simulink model "Vehicle_Dynamics_Tests"  (R2013b)
settings: Solver=ode15s  StartTime=0.0  StopTime=10  MaxStep=0.01  RelTol=1e-4  AbsTol=1e-4
PostLoadFcn:
  | Configure_TNO_Tire_Test('handling');
undefined symbols (not defined in the file or in its folder): angparking, delta, is, TNO_Veh_PARAM, tparking, tswd, tvxset, vxset, X, Y, Z
libraries: sm_lib x53, nesl_utility x25, Delft_Tyre_sm2glib x16
(part 1 of 2)
Description:
  | Copyright 2013 The MathWorks, Inc.
settings Model: Creator=smiller  LastModifiedBy=hofstadrhmtvd
settings DataIOCC: LimitDataPoints=off  SaveOutput=off  OutputTimes=[0:0.01:10]
settings OptimizationCC: ExpressionDepthLimit=2147483647
settings DebuggingCC: StateNameClashWarn=warning
settings ConfigurationSet: Description=SimMechanics 2G
settings ExplorerConfigSet: InternalSimMechanicsExplorerSettings="<ExplorerConfiguration><canonicalview>default</canonicalview><TilePanel><TileInfo><Tiles Columns=\"1\" Count=\"1\" Rows=\"1\"><Column Left=\"2\" Weight=\"1\"/><Column Left=\"786\"/><Row Top=\"2\" Weight=\"1\"/><Row Top=\"392\"/><Tile Height=\"1\" Width=\"1\" X=\"0\" Y=\"0\"/></Tiles></TileInfo><SceneInfo><SceneViewer><BGColor><R>0.80000001192092896</R><G>0.80000001192092896</G><B>0.80000001192092896</B></BGColor><Camera><Position><X>5.6749032986341916</X><Y>0.8952491746014456</Y><Z>0.76840563569508813</Z></Position><Center><X>-1.5032858848571777</X><Y>0.8952491746014456</Y><Z>0.76840563569508813</Z></Center><Up><X>-0</X><Y>0</Y><Z>1</Z></Up><Left>-1.4372989570944883</Left><Right>1.4372989570944883</Right><Bottom>-1.1681998313418454</Bottom><Top>1.1681998313418454</Top></Camera></SceneViewer></SceneInfo></TilePanel></ExplorerConfiguration>"

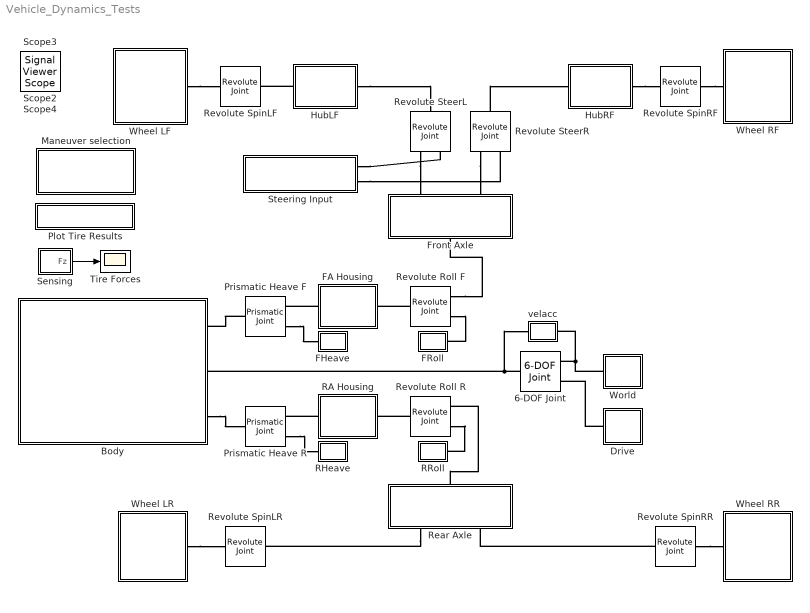
== system Vehicle_Dynamics_Tests ==
  6-DOF Joint : sm_lib/Joints/6-DOF Joint  SenseConstraintForceX=off  SenseConstraintForceY=off  SenseConstraintForceZ=off  SenseConstraintTorqueX=off  SenseConstraintTorqueY=off  SenseConstraintTorqueZ=off  ConstraintWrenchDir=FollowerOnBase  ConstraintWrenchFrame=BaseFrame  PxEquilibriumPosition=0  PxEquilibriumPositionUnits=m  PxSpringStiffness=0  PxSpringStiffnessUnits=N/m  PxDampingCoefficient=0  PxDampingCoefficientUnits=N/(m/s)  PxTorqueActuationMode=InputTorque  PxMotionActuationMode=ComputedMotion  PxSensePosition=off  PxSenseVelocity=off  PxSenseAcceleration=off  PxSenseTorqueForce=off  PxPositionTargetValue=0  PxPositionTargetValueUnits=m  PxPositionTargetSpecify=off  PxPositionTargetPriority=High  PxVelocityTargetValue=TNO_Veh_PARAM.InitVel.Vehicle  PxVelocityTargetValueUnits=m/s  PxVelocityTargetSpecify=on  PxVelocityTargetPriority=High  PyEquilibriumPosition=0  PyEquilibriumPositionUnits=m  PySpringStiffness=0  PySpringStiffnessUnits=N/m  PyDampingCoefficient=0  PyDampingCoefficientUnits=N/(m/s)  PyTorqueActuationMode=NoTorque  PyMotionActuationMode=ComputedMotion  PySensePosition=off  PySenseVelocity=off  PySenseAcceleration=off  PySenseTorqueForce=off  PyPositionTargetValue=0  PyPositionTargetValueUnits=m  PyPositionTargetSpecify=off  PyPositionTargetPriority=High  PyVelocityTargetValue=0  PyVelocityTargetValueUnits=m/s  PyVelocityTargetSpecify=off  PyVelocityTargetPriority=High  PzEquilibriumPosition=0  PzEquilibriumPositionUnits=m  PzSpringStiffness=0  PzSpringStiffnessUnits=N/m  PzDampingCoefficient=0  PzDampingCoefficientUnits=N/(m/s)  PzTorqueActuationMode=NoTorque  PzMotionActuationMode=ComputedMotion  PzSensePosition=off  PzSenseVelocity=off  PzSenseAcceleration=off  PzSenseTorqueForce=off  PzPositionTargetValue=0  PzPositionTargetValueUnits=m  PzPositionTargetSpecify=off  PzPositionTargetPriority=High  PzVelocityTargetValue=0  PzVelocityTargetValueUnits=m/s  PzVelocityTargetSpecify=off  PzVelocityTargetPriority=High  SphDefPosRotationMethod=None  SphDefPosRotationAngleUnits=deg  SphDefPosRotationStandardAxis=+Z  SphDefPosRotationAngle=0  SphDefPosRotationArbitraryAxis=[0 0 1]  SphDefPosFollAlignAxisA=+X  SphDefPosBaseAlignAxisA=+Y  SphDefPosFollAlignAxisB=+Y  SphDefPosBaseAlignAxisB=+Z  SphEqPosRotationMethod=None  SphEqPosRotationAngleUnits=deg  SphEqPosRotationStandardAxis=+Z  SphEqPosRotationAngle=0  SphEqPosRotationArbitraryAxis=[0 0 1]  SphEqPosFollAlignAxisA=+X  SphEqPosBaseAlignAxisA=+Y  SphEqPosFollAlignAxisB=+Y  SphEqPosBaseAlignAxisB=+Z  SphSpringStiffness=0  SphSpringStiffnessUnits=N*m/deg  SphDampingCoefficient=0  SphDampingCoefficientUnits=N*m/(deg/s)  SphActuateTorqueX=off  SphActuateTorqueY=off  SphActuateTorqueZ=off  SphActuateTorque=off  SphTorqueActuationMode=NoTorque  SphMotionActuationMode=ComputedMotion  SphActuationFrame=BaseFrame  SphSensePosition=off  SphSenseVelocityX=off  SphSenseVelocityY=off  SphSenseVelocityZ=off  SphSenseVelocity=off  SphSenseAccelerationX=off  SphSenseAccelerationY=off  SphSenseAccelerationZ=off  SphSenseAcceleration=off  SphSenseTorqueX=off  SphSenseTorqueY=off  SphSenseTorqueZ=off  SphSenseTorqueForce=off  SphSensingFrame=BaseFrame  SphPositionTargetRotationMethod=None  SphPositionTargetRotationAngleUnits=deg  SphPositionTargetRotationStandardAxis=+Z  SphPositionTargetRotationAngle=0  SphPositionTargetRotationArbitraryAxis=[0 0 1]  SphPositionTargetFollAlignAxisA=+X  SphPositionTargetBaseAlignAxisA=+Y  SphPositionTargetFollAlignAxisB=+Y  SphPositionTargetBaseAlignAxisB=+Z  SphPositionTargetSpecify=off  SphPositionTargetPriority=High  SphVelocityTargetValue=[0 0 0]  SphVelocityTargetValueUnits=deg/s  SphVelocityTargetSpecify=off  SphVelocityTargetPriority=High  SphVelocityTargetInFollowerFrame=on  BlockFunction=simmechanics.library.joints.sixdof_joint
  Body : Subsystem
      mask Display: image('VehicleBody.png')
  Drive : Subsystem
  FA Housing : Subsystem
  FHeave : Subsystem
      mask Display: disp('FHe');
  FRoll : Subsystem
      mask Display: disp('FRo');
  Front Axle : Subsystem
  HubLF : Subsystem
  HubRF : Subsystem
  Maneuver selection : Subsystem  mask{maneuver_type=Slalom}
      mask prompts: maneuver_type "Maneuver choice"
      mask init:
      | if strcmp(maneuver_type,'Slalom')
      |     Configure_TNO_Tire_Test('slalom');
      | elseif strcmp(maneuver_type,'4 Post Testrig')
      |     Configure_TNO_Tire_Test('4poster');
      | elseif strcmp(maneuver_type,'Parking')
      |     Configure_TNO_Tire_Test('parking');
      | elseif strcmp(maneuver_type,'Ride')
      |     Configure_TNO_Tire_Test('ride');
      | elseif strcmp(maneuver_type,'Step Steer')
      |     Configure_TNO_Tire_Test('handling');
      | elseif strcmp(maneuver_type,'Sine with Dwell')
      |     Configure_TNO_Tire_Test('sinewithdwell');
      | end
      mask TypeOptions maneuver_type: Slalom | 4 Post Testrig | Parking | Ride | Step Steer | Sine with Dwell
      mask DialogControl Update_Diagram Prompt: Update Diagram
      mask DialogControl Update_Diagram Callback: set_param(bdroot,'SimulationCommand','Update')
      mask Display:
      | fprintf('Maneuver:\n\n')
      | fprintf(maneuver_type);
  Plot Tire Results : Subsystem
      settings: OpenFcn=PlotTireOutputs_UI
      mask Display: disp('Plot Tire Results');
  Prismatic Heave F : sm_lib/Joints/Prismatic Joint  SenseConstraintForceX=off  SenseConstraintForceY=off  SenseConstraintForceZ=off  SenseConstraintTorqueX=off  SenseConstraintTorqueY=off  SenseConstraintTorqueZ=off  ConstraintWrenchDir=FollowerOnBase  ConstraintWrenchFrame=BaseFrame  EquilibriumPosition=TNO_Veh_PARAM.Suspension.FA.Heave.EqPos  EquilibriumPositionUnits=m  SpringStiffness=TNO_Veh_PARAM.Suspension.FA.Heave.Stiffness  SpringStiffnessUnits=N/m  DampingCoefficient=TNO_Veh_PARAM.Suspension.FA.Heave.Damping  DampingCoefficientUnits=N/(m/s)  TorqueActuationMode=NoTorque  MotionActuationMode=ComputedMotion  SensePosition=on  SenseVelocity=off  SenseAcceleration=off  SenseTorqueForce=off  PositionTargetValue=0  PositionTargetValueUnits=m  PositionTargetSpecify=off  PositionTargetPriority=High  VelocityTargetValue=0  VelocityTargetValueUnits=m/s  VelocityTargetSpecify=off  VelocityTargetPriority=High  BlockFunction=simmechanics.library.joints.prismatic_joint
  Prismatic Heave R : sm_lib/Joints/Prismatic Joint  SenseConstraintForceX=off  SenseConstraintForceY=off  SenseConstraintForceZ=off  SenseConstraintTorqueX=off  SenseConstraintTorqueY=off  SenseConstraintTorqueZ=off  ConstraintWrenchDir=FollowerOnBase  ConstraintWrenchFrame=BaseFrame  EquilibriumPosition=TNO_Veh_PARAM.Suspension.RA.Heave.EqPos  EquilibriumPositionUnits=m  SpringStiffness=TNO_Veh_PARAM.Suspension.RA.Heave.Stiffness  SpringStiffnessUnits=N/m  DampingCoefficient=TNO_Veh_PARAM.Suspension.RA.Heave.Damping  DampingCoefficientUnits=N/(m/s)  TorqueActuationMode=NoTorque  MotionActuationMode=ComputedMotion  SensePosition=on  SenseVelocity=off  SenseAcceleration=off  SenseTorqueForce=off  PositionTargetValue=0  PositionTargetValueUnits=m  PositionTargetSpecify=off  PositionTargetPriority=High  VelocityTargetValue=0  VelocityTargetValueUnits=m/s  VelocityTargetSpecify=off  VelocityTargetPriority=High  BlockFunction=simmechanics.library.joints.prismatic_joint
  RA Housing : Subsystem
  RHeave : Subsystem
      mask Display: disp('RHe')
  RRoll : Subsystem
      mask Display: disp('RRo');
  Rear Axle : Subsystem
  Revolute SpinLF : sm_lib/Joints/Revolute Joint  SenseConstraintForceX=off  SenseConstraintForceY=off  SenseConstraintForceZ=off  SenseConstraintTorqueX=off  SenseConstraintTorqueY=off  SenseConstraintTorqueZ=off  ConstraintWrenchDir=FollowerOnBase  ConstraintWrenchFrame=BaseFrame  EquilibriumPosition=0  EquilibriumPositionUnits=rad  SpringStiffness=0  SpringStiffnessUnits=N*m/rad  DampingCoefficient=0  DampingCoefficientUnits=N*m/(rad/s)  TorqueActuationMode=NoTorque  MotionActuationMode=ComputedMotion  SensePosition=off  SenseVelocity=off  SenseAcceleration=off  SenseTorqueForce=off  PositionTargetValue=0  PositionTargetValueUnits=deg  PositionTargetSpecify=off  PositionTargetPriority=High  VelocityTargetValue=TNO_Veh_PARAM.InitVel.LF  VelocityTargetValueUnits=rad/s  VelocityTargetSpecify=on  VelocityTargetPriority=High  BlockFunction=simmechanics.library.joints.revolute_joint
  Revolute SpinLR : sm_lib/Joints/Revolute Joint  SenseConstraintForceX=off  SenseConstraintForceY=off  SenseConstraintForceZ=off  SenseConstraintTorqueX=off  SenseConstraintTorqueY=off  SenseConstraintTorqueZ=off  ConstraintWrenchDir=FollowerOnBase  ConstraintWrenchFrame=BaseFrame  EquilibriumPosition=0  EquilibriumPositionUnits=rad  SpringStiffness=0  SpringStiffnessUnits=N*m/rad  DampingCoefficient=0  DampingCoefficientUnits=N*m/(rad/s)  TorqueActuationMode=NoTorque  MotionActuationMode=ComputedMotion  SensePosition=off  SenseVelocity=off  SenseAcceleration=off  SenseTorqueForce=off  PositionTargetValue=0  PositionTargetValueUnits=deg  PositionTargetSpecify=off  PositionTargetPriority=High  VelocityTargetValue=TNO_Veh_PARAM.InitVel.LR  VelocityTargetValueUnits=rad/s  VelocityTargetSpecify=on  VelocityTargetPriority=High  BlockFunction=simmechanics.library.joints.revolute_joint
  Revolute SpinRF : sm_lib/Joints/Revolute Joint  SenseConstraintForceX=off  SenseConstraintForceY=off  SenseConstraintForceZ=off  SenseConstraintTorqueX=off  SenseConstraintTorqueY=off  SenseConstraintTorqueZ=off  ConstraintWrenchDir=FollowerOnBase  ConstraintWrenchFrame=BaseFrame  EquilibriumPosition=0  EquilibriumPositionUnits=rad  SpringStiffness=0  SpringStiffnessUnits=N*m/rad  DampingCoefficient=0  DampingCoefficientUnits=N*m/(rad/s)  TorqueActuationMode=NoTorque  MotionActuationMode=ComputedMotion  SensePosition=off  SenseVelocity=off  SenseAcceleration=off  SenseTorqueForce=off  PositionTargetValue=0  PositionTargetValueUnits=deg  PositionTargetSpecify=off  PositionTargetPriority=High  VelocityTargetValue=TNO_Veh_PARAM.InitVel.RF  VelocityTargetValueUnits=rad/s  VelocityTargetSpecify=on  VelocityTargetPriority=High  BlockFunction=simmechanics.library.joints.revolute_joint
  Revolute SpinRR : sm_lib/Joints/Revolute Joint  SenseConstraintForceX=off  SenseConstraintForceY=off  SenseConstraintForceZ=off  SenseConstraintTorqueX=off  SenseConstraintTorqueY=off  SenseConstraintTorqueZ=off  ConstraintWrenchDir=FollowerOnBase  ConstraintWrenchFrame=BaseFrame  EquilibriumPosition=0  EquilibriumPositionUnits=rad  SpringStiffness=0  SpringStiffnessUnits=N*m/rad  DampingCoefficient=0  DampingCoefficientUnits=N*m/(rad/s)  TorqueActuationMode=NoTorque  MotionActuationMode=ComputedMotion  SensePosition=off  SenseVelocity=off  SenseAcceleration=off  SenseTorqueForce=off  PositionTargetValue=0  PositionTargetValueUnits=deg  PositionTargetSpecify=off  PositionTargetPriority=High  VelocityTargetValue=TNO_Veh_PARAM.InitVel.RR  VelocityTargetValueUnits=rad/s  VelocityTargetSpecify=on  VelocityTargetPriority=High  BlockFunction=simmechanics.library.joints.revolute_joint
  Revolute SteerL : sm_lib/Joints/Revolute Joint  SenseConstraintForceX=off  SenseConstraintForceY=off  SenseConstraintForceZ=off  SenseConstraintTorqueX=off  SenseConstraintTorqueY=off  SenseConstraintTorqueZ=off  ConstraintWrenchDir=FollowerOnBase  ConstraintWrenchFrame=BaseFrame  EquilibriumPosition=0  EquilibriumPositionUnits=rad  SpringStiffness=0  SpringStiffnessUnits=N*m/rad  DampingCoefficient=0  DampingCoefficientUnits=N*m/(rad/s)  TorqueActuationMode=ComputedTorque  MotionActuationMode=InputMotion  SensePosition=off  SenseVelocity=off  SenseAcceleration=off  SenseTorqueForce=off  PositionTargetValue=0  PositionTargetValueUnits=deg  PositionTargetSpecify=off  PositionTargetPriority=High  VelocityTargetValue=66  VelocityTargetValueUnits=rad/s  VelocityTargetSpecify=off  VelocityTargetPriority=High  BlockFunction=simmechanics.library.joints.revolute_joint
  Revolute SteerR : sm_lib/Joints/Revolute Joint  SenseConstraintForceX=off  SenseConstraintForceY=off  SenseConstraintForceZ=off  SenseConstraintTorqueX=off  SenseConstraintTorqueY=off  SenseConstraintTorqueZ=off  ConstraintWrenchDir=FollowerOnBase  ConstraintWrenchFrame=BaseFrame  EquilibriumPosition=0  EquilibriumPositionUnits=rad  SpringStiffness=0  SpringStiffnessUnits=N*m/rad  DampingCoefficient=0  DampingCoefficientUnits=N*m/(rad/s)  TorqueActuationMode=ComputedTorque  MotionActuationMode=InputMotion  SensePosition=off  SenseVelocity=off  SenseAcceleration=off  SenseTorqueForce=off  PositionTargetValue=0  PositionTargetValueUnits=deg  PositionTargetSpecify=off  PositionTargetPriority=High  VelocityTargetValue=66  VelocityTargetValueUnits=rad/s  VelocityTargetSpecify=off  VelocityTargetPriority=High  BlockFunction=simmechanics.library.joints.revolute_joint
  Revolute Roll F : sm_lib/Joints/Revolute Joint  SenseConstraintForceX=off  SenseConstraintForceY=off  SenseConstraintForceZ=off  SenseConstraintTorqueX=off  SenseConstraintTorqueY=off  SenseConstraintTorqueZ=off  ConstraintWrenchDir=FollowerOnBase  ConstraintWrenchFrame=BaseFrame  EquilibriumPosition=0  EquilibriumPositionUnits=rad  SpringStiffness=TNO_Veh_PARAM.Suspension.FA.Roll.Stiffness  SpringStiffnessUnits=N*m/rad  DampingCoefficient=TNO_Veh_PARAM.Suspension.FA.Roll.Damping  DampingCoefficientUnits=N*m/(rad/s)  TorqueActuationMode=NoTorque  MotionActuationMode=ComputedMotion  SensePosition=on  SenseVelocity=off  SenseAcceleration=off  SenseTorqueForce=off  PositionTargetValue=0  PositionTargetValueUnits=deg  PositionTargetSpecify=off  PositionTargetPriority=High  VelocityTargetValue=0  VelocityTargetValueUnits=deg/s  VelocityTargetSpecify=off  VelocityTargetPriority=High  BlockFunction=simmechanics.library.joints.revolute_joint
  Revolute Roll R : sm_lib/Joints/Revolute Joint  SenseConstraintForceX=off  SenseConstraintForceY=off  SenseConstraintForceZ=off  SenseConstraintTorqueX=off  SenseConstraintTorqueY=off  SenseConstraintTorqueZ=off  ConstraintWrenchDir=FollowerOnBase  ConstraintWrenchFrame=BaseFrame  EquilibriumPosition=0  EquilibriumPositionUnits=rad  SpringStiffness=TNO_Veh_PARAM.Suspension.RA.Roll.Stiffness  SpringStiffnessUnits=N*m/rad  DampingCoefficient=TNO_Veh_PARAM.Suspension.RA.Roll.Damping  DampingCoefficientUnits=N*m/(rad/s)  TorqueActuationMode=NoTorque  MotionActuationMode=ComputedMotion  SensePosition=on  SenseVelocity=off  SenseAcceleration=off  SenseTorqueForce=off  PositionTargetValue=0  PositionTargetValueUnits=deg  PositionTargetSpecify=off  PositionTargetPriority=High  VelocityTargetValue=0  VelocityTargetValueUnits=deg/s  VelocityTargetSpecify=off  VelocityTargetPriority=High  BlockFunction=simmechanics.library.joints.revolute_joint
  Sensing : Subsystem
  Steering Input : Subsystem  Variant=on  OverrideUsingVariant=Slalom
  Tire Forces : Scope
      settings: YMin=3500  YMax=6000
  Wheel LF : Subsystem
      mask Display: image('WheelL.png')
  Wheel LR : Subsystem
      mask Display: image('WheelL.png')
  Wheel RF : Subsystem
      mask Display: image('WheelR.png')
  Wheel RR : Subsystem
      mask Display: image('WheelR.png')
  World : Subsystem
  velacc : Subsystem
      mask Display: disp('va')
  Scope2 : SignalViewerScope  IOType=viewer  RefreshTime=0.035000
  Scope3 : SignalViewerScope  IOType=viewer  ZoomMode=yonly  LegendLocations="0.77309     0.66156     0.17615     0.19796"  RefreshTime=0.035000
      settings: ShowLegends=on
  Scope4 : SignalViewerScope  IOType=viewer  RefreshTime=0.035000
      settings: SaveName=ScopeData2
  wires:
  Sensing/1(Fz) -> Tire Forces/1
  connections:
  6-DOF Joint/RConn1 -- velacc/RConn1 -- Body/LConn2
  World/LConn1 -- velacc/LConn1 -- 6-DOF Joint/LConn1
  Rear Axle/RConn1 -- Revolute SpinLR/LConn1
  Revolute SteerR/LConn1 -- Front Axle/RConn2
  Revolute SteerL/LConn1 -- Front Axle/RConn1
  Steering Input/RConn1 -- Revolute SteerL/LConn2
  Prismatic Heave F/LConn1 -- Body/LConn1
  Revolute Roll F/RConn1 -- Front Axle/LConn1
  Revolute Roll R/LConn1 -- RA Housing/RConn1
  Rear Axle/LConn1 -- Revolute Roll R/RConn1
  Body/LConn3 -- Prismatic Heave R/LConn1
  RA Housing/LConn1 -- Prismatic Heave R/RConn1
  FA Housing/LConn1 -- Prismatic Heave F/RConn1
  Revolute Roll F/LConn1 -- FA Housing/RConn1
  Prismatic Heave F/RConn2 -- FHeave/RConn1
  Revolute Roll F/RConn2 -- FRoll/RConn1
  Prismatic Heave R/RConn2 -- RHeave/LConn1
  Revolute Roll R/RConn2 -- RRoll/RConn1
  HubLF/LConn1 -- Revolute SteerL/RConn1
  HubLF/RConn1 -- Revolute SpinLF/LConn1
  HubRF/RConn1 -- Revolute SpinRF/LConn1
  Revolute SpinRF/RConn1 -- Wheel RF/LConn1
  Revolute SpinRR/RConn1 -- Wheel RR/LConn1
  Wheel LR/RConn1 -- Revolute SpinLR/RConn1
  Wheel LF/RConn1 -- Revolute SpinLF/RConn1
  Revolute SteerR/RConn1 -- HubRF/LConn1
  Revolute SpinRR/LConn1 -- Rear Axle/RConn2
  Steering Input/RConn2 -- Revolute SteerR/LConn2
  Drive/LConn1 -- 6-DOF Joint/LConn2

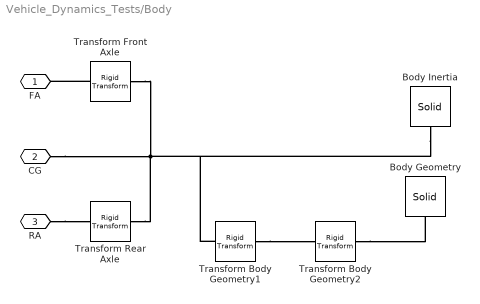
== system Vehicle_Dynamics_Tests/Body ==
  Body Geometry : sm_lib/Body Elements/Solid  InertiaType=Custom  Mass=0  MassUnits=kg  CenterOfMass=[0 0 0]  CenterOfMassUnits=m  MomentsOfInertia=[0 0 0]  MomentsOfInertiaUnits=kg*m^2  ProductsOfInertia=[0 0 0]  ProductsOfInertiaUnits=kg*m^2  DensityBased=on  Density=1000  DensityUnits=kg/(m^3)  GraphicType=FromGeometry  MarkerShape=Sphere  MarkerSize=10  MarkerSizeUnits=m  GraphicVisPropType=SimpleVisualProperties  GraphicDiffuseColor=[0.6 0.8 1.0]  GraphicSpecularColor=[0.5 0.5 0.5 1.0]  GraphicAmbientColor=[0.15 0.15 0.15 1.0]  GraphicEmissiveColor=[0.0 0.0 0.0 1.0]  GraphicShininess=75  GraphicOpacity=1  GeometryShape=FromFile  RectangleSize=[1 1]  RectangleSizeUnits=m  BrickDimensions=TNO_Veh_PARAM.Body.LWH  BrickDimensionUnits=m  CylinderRadius=1  CylinderRadiusUnits=m  CylinderLength=1  CylinderLengthUnits=m  SphereRadius=1  SphereRadiusUnits=m  EllipsoidRadii=[1 1 1]  EllipsoidRadiiUnits=m  ExtrusionCrossSection=[1 1; -1 1; -1 -1; 1 -1]  ExtrusionCrossSectionUnits=m  ExtrusionLength=1  ExtrusionLengthUnits=m  PolygonNumSides=3  PolygonOuterRadius=1  PolygonOuterRadiusUnits=m  ExtGeomFileName=VehicleBody.STL  ExtGeomFileUnits=mm  RevolutionCrossSection=[1 1; 1 -1; 2 -1; 2 1]  RevolutionCrossSectionUnits=m  RevolutionExtent=Full  RevolutionAngle=180  RevolutionAngleUnits=deg  BlockFunction=simmechanics.library.body_elements.solid
  Body Inertia : sm_lib/Body Elements/Solid  InertiaType=Custom  Mass=TNO_Veh_PARAM.Body.Mass  MassUnits=kg  CenterOfMass=[0 0 0]  CenterOfMassUnits=m  MomentsOfInertia=TNO_Veh_PARAM.Body.Inertias  MomentsOfInertiaUnits=kg*m^2  ProductsOfInertia=[0 0 0]  ProductsOfInertiaUnits=kg*m^2  DensityBased=on  Density=1000  DensityUnits=kg/(m^3)  GraphicType=FromGeometry  MarkerShape=Sphere  MarkerSize=10  MarkerSizeUnits=m  GraphicVisPropType=SimpleVisualProperties  GraphicDiffuseColor=[0.4 0.6 1.0]  GraphicSpecularColor=[0.5 0.5 0.5 1.0]  GraphicAmbientColor=[0.15 0.15 0.15 1.0]  GraphicEmissiveColor=[0.0 0.0 0.0 1.0]  GraphicShininess=75  GraphicOpacity=1.0  GeometryShape=Brick  RectangleSize=[1 1]  RectangleSizeUnits=m  BrickDimensions=TNO_Veh_PARAM.Body.LWH  BrickDimensionUnits=m  CylinderRadius=1  CylinderRadiusUnits=m  CylinderLength=1  CylinderLengthUnits=m  SphereRadius=1  SphereRadiusUnits=m  EllipsoidRadii=[1 1 1]  EllipsoidRadiiUnits=m  ExtrusionCrossSection=[1 1; -1 1; -1 -1; 1 -1]  ExtrusionCrossSectionUnits=m  ExtrusionLength=1  ExtrusionLengthUnits=m  PolygonNumSides=3  PolygonOuterRadius=1  PolygonOuterRadiusUnits=m  ExtGeomFileName=L:\PhysModDevTeamProject\MF_Tyre_64b\Demos\SimMechanics_demos\CadImportFiles\BMW M3-IGS - Imported1-1.STL  ExtGeomFileUnits=mm  RevolutionCrossSection=[1 1; 1 -1; 2 -1; 2 1]  RevolutionCrossSectionUnits=m  RevolutionExtent=Full  RevolutionAngle=180  RevolutionAngleUnits=deg  BlockFunction=simmechanics.library.body_elements.solid
  Transform Front Axle : sm_lib/Frames and Transforms/Rigid Transform  TranslationMethod=Cartesian  TranslationLengthUnit=m  TranslationStandardAxis=+Z  TranslationStandardOffset=0  TranslationCartesianOffset=[TNO_Veh_PARAM.Body.Length/2 0 -TNO_Veh_PARAM.Suspension.FA.Heave.Height]  TranslationROffset=0  TranslationROffsetUnits=m  TranslationZOffset=0  TranslationZOffsetUnits=m  TranslationThetaOffset=0  TranslationThetaOffsetUnits=deg  RotationMethod=None  RotationAngleUnits=deg  RotationStandardAxis=+Z  RotationAngle=0  RotationArbitraryAxis=[0 0 1]  FollAlignAxisA=+X  BaseAlignAxisA=+Y  FollAlignAxisB=+Y  BaseAlignAxisB=+Z  BlockFunction=simmechanics.library.frames_transforms.rigid_transform
  Transform Rear Axle : sm_lib/Frames and Transforms/Rigid Transform  TranslationMethod=Cartesian  TranslationLengthUnit=m  TranslationStandardAxis=+Z  TranslationStandardOffset=0  TranslationCartesianOffset=[-TNO_Veh_PARAM.Body.Length/2 0 -TNO_Veh_PARAM.Suspension.RA.Heave.Height]  TranslationROffset=0  TranslationROffsetUnits=m  TranslationZOffset=0  TranslationZOffsetUnits=m  TranslationThetaOffset=0  TranslationThetaOffsetUnits=deg  RotationMethod=None  RotationAngleUnits=deg  RotationStandardAxis=+Z  RotationAngle=0  RotationArbitraryAxis=[0 0 1]  FollAlignAxisA=+X  BaseAlignAxisA=+Y  FollAlignAxisB=+Y  BaseAlignAxisB=+Z  BlockFunction=simmechanics.library.frames_transforms.rigid_transform
  Transform Body Geometry1 : sm_lib/Frames and Transforms/Rigid Transform  TranslationMethod=None  TranslationLengthUnit=m  TranslationStandardAxis=+Z  TranslationStandardOffset=0  TranslationCartesianOffset=TNO_Veh_PARAM.Body.GraphicsShift  TranslationROffset=0  TranslationROffsetUnits=m  TranslationZOffset=0  TranslationZOffsetUnits=m  TranslationThetaOffset=0  TranslationThetaOffsetUnits=deg  RotationMethod=StandardAxis  RotationAngleUnits=deg  RotationStandardAxis=-Z  RotationAngle=90  RotationArbitraryAxis=[0 0 1]  FollAlignAxisA=+X  BaseAlignAxisA=+Y  FollAlignAxisB=+Y  BaseAlignAxisB=+Z  BlockFunction=simmechanics.library.frames_transforms.rigid_transform
  Transform Body Geometry2 : sm_lib/Frames and Transforms/Rigid Transform  TranslationMethod=Cartesian  TranslationLengthUnit=m  TranslationStandardAxis=+Z  TranslationStandardOffset=0  TranslationCartesianOffset=TNO_Veh_PARAM.Body.GraphicsShift  TranslationROffset=0  TranslationROffsetUnits=m  TranslationZOffset=0  TranslationZOffsetUnits=m  TranslationThetaOffset=0  TranslationThetaOffsetUnits=deg  RotationMethod=StandardAxis  RotationAngleUnits=deg  RotationStandardAxis=+X  RotationAngle=90  RotationArbitraryAxis=[0 0 1]  FollAlignAxisA=+X  BaseAlignAxisA=+Y  FollAlignAxisB=+Y  BaseAlignAxisB=+Z  BlockFunction=simmechanics.library.frames_transforms.rigid_transform
  FA : PMIOPort  Port=1  Side=Left
  CG : PMIOPort  Port=2  Side=Left
  RA : PMIOPort  Port=3  Side=Left
  connections:
  Transform Front Axle/RConn1 -- FA/RConn1
  RA/RConn1 -- Transform Rear Axle/RConn1
  Transform Rear Axle/LConn1 -- Transform Front Axle/LConn1 -- Body Inertia/RConn1 -- Transform Body Geometry1/LConn1 -- CG/RConn1
  Transform Body Geometry2/RConn1 -- Body Geometry/RConn1
  Transform Body Geometry1/RConn1 -- Transform Body Geometry2/LConn1

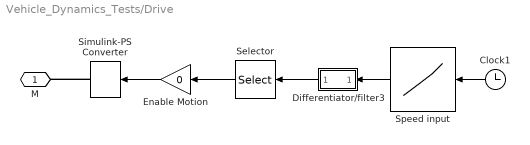
== system Vehicle_Dynamics_Tests/Drive ==
  Clock1 : Clock
  Differentiator/filter3 : Subsystem  mask{ts=0.05}
      mask prompts: ts "response_time"
      mask init:
      | c=(3*pi/ts)^2;
  Enable Motion : Gain  Gain=0
  Selector : Selector  InputPortWidth=3  IndexOptions=Index vector (dialog)  Indices=[1]  OutputSizes=1
  Simulink-PS Converter : nesl_utility/Simulink-PS Converter  PhysicalDomain=network_engine_domain  SubClassName=ps_input  LeftPortType=input  RightPortType=output  PseudoPeriodic=off  Frequencies=[]  NoiseDistribution=none  NoiseParameters=[]  Unit=1  AffineConversion=off  InputFiltering=on  SimscapeFilterOrder=2  InputFilterTimeConstant=0.001  UdotUserProvided=1
  Speed input : Lookup  InputValues=tvxset  Table=vxset
  M : PMIOPort  Port=1  Side=Left
  wires:
  Selector/1 -> Enable Motion/1
  Differentiator/filter3/1(Out2) -> Selector/1
  Clock1/1 -> Speed input/1
  Speed input/1 -> Differentiator/filter3/1(In2)
  Enable Motion/1 -> Simulink-PS Converter/1
  connections:
  Simulink-PS Converter/RConn1 -- M/RConn1

== system Vehicle_Dynamics_Tests/FA Housing ==
  Axle Ctr : sm_lib/Body Elements/Solid  InertiaType=CalculateFromGeometry  Mass=1  MassUnits=kg  CenterOfMass=[0 0 0]  CenterOfMassUnits=m  MomentsOfInertia=[1 1 1]  MomentsOfInertiaUnits=kg*m^2  ProductsOfInertia=[0 0 0]  ProductsOfInertiaUnits=kg*m^2  DensityBased=on  Density=1000  DensityUnits=kg/(m^3)  GraphicType=FromGeometry  MarkerShape=Sphere  MarkerSize=10  MarkerSizeUnits=m  GraphicVisPropType=SimpleVisualProperties  GraphicDiffuseColor=[0.6 0.6 0.6]  GraphicSpecularColor=[0.5 0.5 0.5 1.0]  GraphicAmbientColor=[0.15 0.15 0.15 1.0]  GraphicEmissiveColor=[0.0 0.0 0.0 1.0]  GraphicShininess=75  GraphicOpacity=1.0  GeometryShape=Cylinder  RectangleSize=[1 1]  RectangleSizeUnits=m  BrickDimensions=[3 1 0.5]  BrickDimensionUnits=m  CylinderRadius=TNO_Veh_PARAM.Axle_Housing.Radius  CylinderRadiusUnits=m  CylinderLength=TNO_Veh_PARAM.Axle_Housing.Length  CylinderLengthUnits=m  SphereRadius=1  SphereRadiusUnits=m  EllipsoidRadii=[1 1 1]  EllipsoidRadiiUnits=m  ExtrusionCrossSection=[1 1; -1 1; -1 -1; 1 -1]  ExtrusionCrossSectionUnits=m  ExtrusionLength=1  ExtrusionLengthUnits=m  PolygonNumSides=3  PolygonOuterRadius=1  PolygonOuterRadiusUnits=m  ExtGeomFileUnits=m  RevolutionCrossSection=[1 1; 1 -1; 2 -1; 2 1]  RevolutionCrossSectionUnits=m  RevolutionExtent=Full  RevolutionAngle=180  RevolutionAngleUnits=deg  BlockFunction=simmechanics.library.body_elements.solid
  Transform (Body) : sm_lib/Frames and Transforms/Rigid Transform  TranslationMethod=None  TranslationLengthUnit=m  TranslationStandardAxis=+Z  TranslationStandardOffset=0  TranslationCartesianOffset=[0 0 0]  TranslationROffset=0  TranslationROffsetUnits=m  TranslationZOffset=0  TranslationZOffsetUnits=m  TranslationThetaOffset=0  TranslationThetaOffsetUnits=deg  RotationMethod=StandardAxis  RotationAngleUnits=deg  RotationStandardAxis=+X  RotationAngle=90  RotationArbitraryAxis=[0 0 1]  FollAlignAxisA=+X  BaseAlignAxisA=+Y  FollAlignAxisB=+Y  BaseAlignAxisB=+Z  BlockFunction=simmechanics.library.frames_transforms.rigid_transform
  Transform (FA) : sm_lib/Frames and Transforms/Rigid Transform  TranslationMethod=StandardAxis  TranslationLengthUnit=m  TranslationStandardAxis=+Y  TranslationStandardOffset=TNO_Veh_PARAM.Suspension.FA.Roll.Height  TranslationCartesianOffset=[0 0 0]  TranslationROffset=0  TranslationROffsetUnits=m  TranslationZOffset=0  TranslationZOffsetUnits=m  TranslationThetaOffset=0  TranslationThetaOffsetUnits=deg  RotationMethod=StandardAxis  RotationAngleUnits=deg  RotationStandardAxis=+Y  RotationAngle=90  RotationArbitraryAxis=[0 0 1]  FollAlignAxisA=+X  BaseAlignAxisA=+Y  FollAlignAxisB=+Y  BaseAlignAxisB=+Z  BlockFunction=simmechanics.library.frames_transforms.rigid_transform
  Body : PMIOPort  Port=1  Side=Left
  FA : PMIOPort  Port=2  Side=Right
  connections:
  Transform (Body)/RConn1 -- Body/RConn1
  Axle Ctr/RConn1 -- Transform (Body)/LConn1 -- Transform (FA)/LConn1
  FA/RConn1 -- Transform (FA)/RConn1

== system Vehicle_Dynamics_Tests/FHeave ==
  PS-Simulink Converter20 : nesl_utility/PS-Simulink Converter  PhysicalDomain=network_engine_domain  SubClassName=ps_output  LeftPortType=input  RightPortType=output  PseudoPeriodic=off  Frequencies=[]  Unit=m  AffineConversion=off
  To Workspace : ToWorkspace  VariableName=FAheave  SampleTime=-1
  Conn1 : PMIOPort  Port=1  Side=Right
  wires:
  PS-Simulink Converter20/1 -> To Workspace/1
  connections:
  Conn1/RConn1 -- PS-Simulink Converter20/LConn1

== system Vehicle_Dynamics_Tests/FRoll ==
  PS-Simulink Converter18 : nesl_utility/PS-Simulink Converter  PhysicalDomain=network_engine_domain  SubClassName=ps_output  LeftPortType=input  RightPortType=output  PseudoPeriodic=off  Frequencies=[]  Unit=deg  AffineConversion=off
  To Workspace1 : ToWorkspace  VariableName=FAroll  SampleTime=-1
  Conn1 : PMIOPort  Port=1  Side=Right
  wires:
  PS-Simulink Converter18/1 -> To Workspace1/1
  connections:
  Conn1/RConn1 -- PS-Simulink Converter18/LConn1

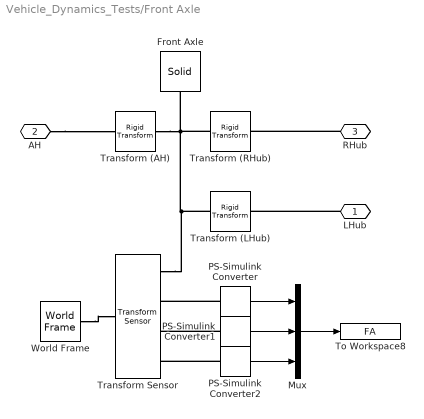
== system Vehicle_Dynamics_Tests/Front Axle ==
  Front Axle : sm_lib/Body Elements/Solid  InertiaType=Custom  Mass=TNO_Veh_PARAM.Axle.FA.Mass  MassUnits=kg  CenterOfMass=[0 0 0]  CenterOfMassUnits=m  MomentsOfInertia=TNO_Veh_PARAM.Axle.FA.Inertia  MomentsOfInertiaUnits=kg*m^2  ProductsOfInertia=[0 0 0]  ProductsOfInertiaUnits=kg*m^2  DensityBased=on  Density=1000  DensityUnits=kg/(m^3)  GraphicType=FromGeometry  MarkerShape=Sphere  MarkerSize=10  MarkerSizeUnits=m  GraphicVisPropType=SimpleVisualProperties  GraphicDiffuseColor=[0.6 0.6 0.6]  GraphicSpecularColor=[0.5 0.5 0.5 1.0]  GraphicAmbientColor=[0.15 0.15 0.15 1.0]  GraphicEmissiveColor=[0.0 0.0 0.0 1.0]  GraphicShininess=75  GraphicOpacity=1.0  GeometryShape=Cylinder  RectangleSize=[1 1]  RectangleSizeUnits=m  BrickDimensions=[3 1 0.5]  BrickDimensionUnits=m  CylinderRadius=TNO_Veh_PARAM.Axle.FA.Radius  CylinderRadiusUnits=m  CylinderLength=TNO_Veh_PARAM.Axle.FA.Length  CylinderLengthUnits=m  SphereRadius=1  SphereRadiusUnits=m  EllipsoidRadii=[1 1 1]  EllipsoidRadiiUnits=m  ExtrusionCrossSection=[1 1; -1 1; -1 -1; 1 -1]  ExtrusionCrossSectionUnits=m  ExtrusionLength=1  ExtrusionLengthUnits=m  PolygonNumSides=3  PolygonOuterRadius=1  PolygonOuterRadiusUnits=m  ExtGeomFileUnits=m  RevolutionCrossSection=[1 1; 1 -1; 2 -1; 2 1]  RevolutionCrossSectionUnits=m  RevolutionExtent=Full  RevolutionAngle=180  RevolutionAngleUnits=deg  BlockFunction=simmechanics.library.body_elements.solid
  Mux : Mux  Inputs=3
  PS-Simulink Converter : nesl_utility/PS-Simulink Converter  PhysicalDomain=network_engine_domain  SubClassName=ps_output  LeftPortType=input  RightPortType=output  PseudoPeriodic=off  Frequencies=[]  Unit=1  AffineConversion=off
  PS-Simulink Converter1 : nesl_utility/PS-Simulink Converter  PhysicalDomain=network_engine_domain  SubClassName=ps_output  LeftPortType=input  RightPortType=output  PseudoPeriodic=off  Frequencies=[]  Unit=1  AffineConversion=off
  PS-Simulink Converter2 : nesl_utility/PS-Simulink Converter  PhysicalDomain=network_engine_domain  SubClassName=ps_output  LeftPortType=input  RightPortType=output  PseudoPeriodic=off  Frequencies=[]  Unit=1  AffineConversion=off
  To Workspace8 : ToWorkspace  VariableName=FA  SampleTime=-1
  Transform (AH) : sm_lib/Frames and Transforms/Rigid Transform  TranslationMethod=StandardAxis  TranslationLengthUnit=m  TranslationStandardAxis=+Y  TranslationStandardOffset=TNO_Veh_PARAM.Axle.FA.Height  TranslationCartesianOffset=[0 0 0]  TranslationROffset=0  TranslationROffsetUnits=m  TranslationZOffset=0  TranslationZOffsetUnits=m  TranslationThetaOffset=0  TranslationThetaOffsetUnits=deg  RotationMethod=StandardAxis  RotationAngleUnits=deg  RotationStandardAxis=+Y  RotationAngle=-90  RotationArbitraryAxis=[0 0 1]  FollAlignAxisA=+X  BaseAlignAxisA=+Y  FollAlignAxisB=+Y  BaseAlignAxisB=+Z  BlockFunction=simmechanics.library.frames_transforms.rigid_transform
  Transform (LHub) : sm_lib/Frames and Transforms/Rigid Transform  TranslationMethod=StandardAxis  TranslationLengthUnit=m  TranslationStandardAxis=+Z  TranslationStandardOffset=-TNO_Veh_PARAM.WheelBase/2  TranslationCartesianOffset=[0 0 0]  TranslationROffset=0  TranslationROffsetUnits=m  TranslationZOffset=0  TranslationZOffsetUnits=m  TranslationThetaOffset=0  TranslationThetaOffsetUnits=deg  RotationMethod=StandardAxis  RotationAngleUnits=deg  RotationStandardAxis=+X  RotationAngle=90  RotationArbitraryAxis=[0 0 1]  FollAlignAxisA=+X  BaseAlignAxisA=+Y  FollAlignAxisB=+Y  BaseAlignAxisB=+Z  BlockFunction=simmechanics.library.frames_transforms.rigid_transform
  Transform (RHub) : sm_lib/Frames and Transforms/Rigid Transform  TranslationMethod=StandardAxis  TranslationLengthUnit=m  TranslationStandardAxis=+Z  TranslationStandardOffset=TNO_Veh_PARAM.WheelBase/2  TranslationCartesianOffset=[0 0 0]  TranslationROffset=0  TranslationROffsetUnits=m  TranslationZOffset=0  TranslationZOffsetUnits=m  TranslationThetaOffset=0  TranslationThetaOffsetUnits=deg  RotationMethod=StandardAxis  RotationAngleUnits=deg  RotationStandardAxis=+X  RotationAngle=90  RotationArbitraryAxis=[0 0 1]  FollAlignAxisA=+X  BaseAlignAxisA=+Y  FollAlignAxisB=+Y  BaseAlignAxisB=+Z  BlockFunction=simmechanics.library.frames_transforms.rigid_transform
  Transform Sensor : sm_lib/Frames and Transforms/Transform Sensor  MeasurementFrame=World  SenseAngle=off  SenseAxis=off  SenseAngle1=off  SenseAngle2=off  SenseAngle3=off  SenseQ=off  SenseR=off  SenseOmegaX=off  SenseOmegaY=off  SenseOmegaZ=off  SenseOmega1=off  SenseOmega2=off  SenseOmega3=off  SenseQDot=off  SenseRDot=off  SenseAlphaX=off  SenseAlphaY=off  SenseAlphaZ=off  SenseAlpha1=off  SenseAlpha2=off  SenseAlpha3=off  SenseQDDot=off  SenseRDDot=off  SenseX=on  SenseY=on  SenseZ=on  SenseRad=off  SenseAzim=off  SenseDist=off  SenseInc=off  SenseXDot=off  SenseYDot=off  SenseZDot=off  SenseRadDot=off  SenseAzimDot=off  SenseDistDot=off  SenseIncDot=off  SenseXDDot=off  SenseYDDot=off  SenseZDDot=off  SenseRadDDot=off  SenseAzimDDot=off  SenseDistDDot=off  SenseIncDDot=off  BlockFunction=simmechanics.library.frames_transforms.transform_sensor
  World Frame : sm_lib/Frames and Transforms/World Frame  BlockFunction=simmechanics.library.frames_transforms.world_frame
  LHub : PMIOPort  Port=1  Side=Right
  AH : PMIOPort  Port=2  Side=Left
  RHub : PMIOPort  Port=3  Side=Right
  wires:
  PS-Simulink Converter/1 -> Mux/1
  PS-Simulink Converter1/1 -> Mux/2
  PS-Simulink Converter2/1 -> Mux/3
  Mux/1 -> To Workspace8/1
  connections:
  LHub/RConn1 -- Transform (LHub)/RConn1
  RHub/RConn1 -- Transform (RHub)/RConn1
  Transform (LHub)/LConn1 -- Transform Sensor/RConn1 -- Front Axle/RConn1 -- Transform (RHub)/LConn1 -- Transform (AH)/LConn1
  AH/RConn1 -- Transform (AH)/RConn1
  World Frame/RConn1 -- Transform Sensor/LConn1
  PS-Simulink Converter1/LConn1 -- Transform Sensor/RConn3
  PS-Simulink Converter/LConn1 -- Transform Sensor/RConn2
  PS-Simulink Converter2/LConn1 -- Transform Sensor/RConn4

== system Vehicle_Dynamics_Tests/HubLF ==
  Hub : sm_lib/Body Elements/Solid  InertiaType=CalculateFromGeometry  Mass=1  MassUnits=kg  CenterOfMass=[0 0 0]  CenterOfMassUnits=m  MomentsOfInertia=[1 1 1]  MomentsOfInertiaUnits=kg*m^2  ProductsOfInertia=[0 0 0]  ProductsOfInertiaUnits=kg*m^2  DensityBased=on  Density=1000  DensityUnits=kg/(m^3)  GraphicType=FromGeometry  MarkerShape=Sphere  MarkerSize=10  MarkerSizeUnits=m  GraphicVisPropType=SimpleVisualProperties  GraphicDiffuseColor=[0.2 0.8 1.0]  GraphicSpecularColor=[0.5 0.5 0.5 1.0]  GraphicAmbientColor=[0.15 0.15 0.15 1.0]  GraphicEmissiveColor=[0.0 0.0 0.0 1.0]  GraphicShininess=75  GraphicOpacity=1.0  GeometryShape=Cylinder  RectangleSize=[1 1]  RectangleSizeUnits=m  BrickDimensions=[3 1 0.5]  BrickDimensionUnits=m  CylinderRadius=TNO_Veh_PARAM.Hub.Radius  CylinderRadiusUnits=m  CylinderLength=TNO_Veh_PARAM.Hub.Length  CylinderLengthUnits=m  SphereRadius=1  SphereRadiusUnits=m  EllipsoidRadii=[1 1 1]  EllipsoidRadiiUnits=m  ExtrusionCrossSection=[1 1; -1 1; -1 -1; 1 -1]  ExtrusionCrossSectionUnits=m  ExtrusionLength=1  ExtrusionLengthUnits=m  PolygonNumSides=3  PolygonOuterRadius=1  PolygonOuterRadiusUnits=m  ExtGeomFileUnits=m  RevolutionCrossSection=[1 1; 1 -1; 2 -1; 2 1]  RevolutionCrossSectionUnits=m  RevolutionExtent=Full  RevolutionAngle=180  RevolutionAngleUnits=deg  BlockFunction=simmechanics.library.body_elements.solid
  Transform (Whl) : sm_lib/Frames and Transforms/Rigid Transform  TranslationMethod=None  TranslationLengthUnit=m  TranslationStandardAxis=+Z  TranslationStandardOffset=0  TranslationCartesianOffset=[0 0 0]  TranslationROffset=0  TranslationROffsetUnits=m  TranslationZOffset=0  TranslationZOffsetUnits=m  TranslationThetaOffset=0  TranslationThetaOffsetUnits=deg  RotationMethod=StandardAxis  RotationAngleUnits=deg  RotationStandardAxis=-X  RotationAngle=90  RotationArbitraryAxis=[0 0 1]  FollAlignAxisA=+X  BaseAlignAxisA=+Y  FollAlignAxisB=+Y  BaseAlignAxisB=+Z  BlockFunction=simmechanics.library.frames_transforms.rigid_transform
  Transform1 (Whl) : sm_lib/Frames and Transforms/Rigid Transform  TranslationMethod=None  TranslationLengthUnit=m  TranslationStandardAxis=+Z  TranslationStandardOffset=0  TranslationCartesianOffset=[0 0 0]  TranslationROffset=0  TranslationROffsetUnits=m  TranslationZOffset=0  TranslationZOffsetUnits=m  TranslationThetaOffset=0  TranslationThetaOffsetUnits=deg  RotationMethod=StandardAxis  RotationAngleUnits=deg  RotationStandardAxis=+Z  RotationAngle=180  RotationArbitraryAxis=[0 0 1]  FollAlignAxisA=+X  BaseAlignAxisA=+Y  FollAlignAxisB=+Y  BaseAlignAxisB=+Z  BlockFunction=simmechanics.library.frames_transforms.rigid_transform
  Axle : PMIOPort  Port=1  Side=Left
  Whl : PMIOPort  Port=2  Side=Right
  connections:
  Transform (Whl)/LConn1 -- Transform1 (Whl)/RConn1
  Transform1 (Whl)/LConn1 -- Axle/RConn1 -- Hub/RConn1
  Whl/RConn1 -- Transform (Whl)/RConn1

== system Vehicle_Dynamics_Tests/HubRF ==
  Hub : sm_lib/Body Elements/Solid  InertiaType=CalculateFromGeometry  Mass=1  MassUnits=kg  CenterOfMass=[0 0 0]  CenterOfMassUnits=m  MomentsOfInertia=[1 1 1]  MomentsOfInertiaUnits=kg*m^2  ProductsOfInertia=[0 0 0]  ProductsOfInertiaUnits=kg*m^2  DensityBased=on  Density=1000  DensityUnits=kg/(m^3)  GraphicType=FromGeometry  MarkerShape=Sphere  MarkerSize=10  MarkerSizeUnits=m  GraphicVisPropType=SimpleVisualProperties  GraphicDiffuseColor=[0.2 0.8 1.0]  GraphicSpecularColor=[0.5 0.5 0.5 1.0]  GraphicAmbientColor=[0.15 0.15 0.15 1.0]  GraphicEmissiveColor=[0.0 0.0 0.0 1.0]  GraphicShininess=75  GraphicOpacity=1.0  GeometryShape=Cylinder  RectangleSize=[1 1]  RectangleSizeUnits=m  BrickDimensions=[3 1 0.5]  BrickDimensionUnits=m  CylinderRadius=TNO_Veh_PARAM.Hub.Radius  CylinderRadiusUnits=m  CylinderLength=TNO_Veh_PARAM.Hub.Length  CylinderLengthUnits=m  SphereRadius=1  SphereRadiusUnits=m  EllipsoidRadii=[1 1 1]  EllipsoidRadiiUnits=m  ExtrusionCrossSection=[1 1; -1 1; -1 -1; 1 -1]  ExtrusionCrossSectionUnits=m  ExtrusionLength=1  ExtrusionLengthUnits=m  PolygonNumSides=3  PolygonOuterRadius=1  PolygonOuterRadiusUnits=m  ExtGeomFileUnits=m  RevolutionCrossSection=[1 1; 1 -1; 2 -1; 2 1]  RevolutionCrossSectionUnits=m  RevolutionExtent=Full  RevolutionAngle=180  RevolutionAngleUnits=deg  BlockFunction=simmechanics.library.body_elements.solid
  Transform (Whl) : sm_lib/Frames and Transforms/Rigid Transform  TranslationMethod=None  TranslationLengthUnit=m  TranslationStandardAxis=+Z  TranslationStandardOffset=0  TranslationCartesianOffset=[0 0 0]  TranslationROffset=0  TranslationROffsetUnits=m  TranslationZOffset=0  TranslationZOffsetUnits=m  TranslationThetaOffset=0  TranslationThetaOffsetUnits=deg  RotationMethod=StandardAxis  RotationAngleUnits=deg  RotationStandardAxis=-X  RotationAngle=90  RotationArbitraryAxis=[0 0 1]  FollAlignAxisA=+X  BaseAlignAxisA=+Y  FollAlignAxisB=+Y  BaseAlignAxisB=+Z  BlockFunction=simmechanics.library.frames_transforms.rigid_transform
  Transform1 (Whl) : sm_lib/Frames and Transforms/Rigid Transform  TranslationMethod=None  TranslationLengthUnit=m  TranslationStandardAxis=+Z  TranslationStandardOffset=0  TranslationCartesianOffset=[0 0 0]  TranslationROffset=0  TranslationROffsetUnits=m  TranslationZOffset=0  TranslationZOffsetUnits=m  TranslationThetaOffset=0  TranslationThetaOffsetUnits=deg  RotationMethod=StandardAxis  RotationAngleUnits=deg  RotationStandardAxis=+Z  RotationAngle=180  RotationArbitraryAxis=[0 0 1]  FollAlignAxisA=+X  BaseAlignAxisA=+Y  FollAlignAxisB=+Y  BaseAlignAxisB=+Z  BlockFunction=simmechanics.library.frames_transforms.rigid_transform
  Axle : PMIOPort  Port=1  Side=Left
  Whl : PMIOPort  Port=2  Side=Right
  connections:
  Hub/RConn1 -- Axle/RConn1 -- Transform1 (Whl)/LConn1
  Transform (Whl)/LConn1 -- Transform1 (Whl)/RConn1
  Whl/RConn1 -- Transform (Whl)/RConn1

== system Vehicle_Dynamics_Tests/Maneuver selection ==

== system Vehicle_Dynamics_Tests/Plot Tire Results ==

== system Vehicle_Dynamics_Tests/RA Housing ==
  Axle Ctr : sm_lib/Body Elements/Solid  InertiaType=CalculateFromGeometry  Mass=1  MassUnits=kg  CenterOfMass=[0 0 0]  CenterOfMassUnits=m  MomentsOfInertia=[1 1 1]  MomentsOfInertiaUnits=kg*m^2  ProductsOfInertia=[0 0 0]  ProductsOfInertiaUnits=kg*m^2  DensityBased=on  Density=1000  DensityUnits=kg/(m^3)  GraphicType=FromGeometry  MarkerShape=Sphere  MarkerSize=10  MarkerSizeUnits=m  GraphicVisPropType=SimpleVisualProperties  GraphicDiffuseColor=[0.6 0.6 0.6]  GraphicSpecularColor=[0.5 0.5 0.5 1.0]  GraphicAmbientColor=[0.15 0.15 0.15 1.0]  GraphicEmissiveColor=[0.0 0.0 0.0 1.0]  GraphicShininess=75  GraphicOpacity=1.0  GeometryShape=Cylinder  RectangleSize=[1 1]  RectangleSizeUnits=m  BrickDimensions=[3 1 0.5]  BrickDimensionUnits=m  CylinderRadius=TNO_Veh_PARAM.Axle_Housing.Radius  CylinderRadiusUnits=m  CylinderLength=TNO_Veh_PARAM.Axle_Housing.Length  CylinderLengthUnits=m  SphereRadius=1  SphereRadiusUnits=m  EllipsoidRadii=[1 1 1]  EllipsoidRadiiUnits=m  ExtrusionCrossSection=[1 1; -1 1; -1 -1; 1 -1]  ExtrusionCrossSectionUnits=m  ExtrusionLength=1  ExtrusionLengthUnits=m  PolygonNumSides=3  PolygonOuterRadius=1  PolygonOuterRadiusUnits=m  ExtGeomFileUnits=m  RevolutionCrossSection=[1 1; 1 -1; 2 -1; 2 1]  RevolutionCrossSectionUnits=m  RevolutionExtent=Full  RevolutionAngle=180  RevolutionAngleUnits=deg  BlockFunction=simmechanics.library.body_elements.solid
  Transform (Body) : sm_lib/Frames and Transforms/Rigid Transform  TranslationMethod=None  TranslationLengthUnit=m  TranslationStandardAxis=+Z  TranslationStandardOffset=0  TranslationCartesianOffset=[0 0.05 0]  TranslationROffset=0  TranslationROffsetUnits=m  TranslationZOffset=0  TranslationZOffsetUnits=m  TranslationThetaOffset=0  TranslationThetaOffsetUnits=deg  RotationMethod=StandardAxis  RotationAngleUnits=deg  RotationStandardAxis=+X  RotationAngle=90  RotationArbitraryAxis=[0 0 1]  FollAlignAxisA=+X  BaseAlignAxisA=+Y  FollAlignAxisB=+Y  BaseAlignAxisB=+Z  BlockFunction=simmechanics.library.frames_transforms.rigid_transform
  Transform (RA) : sm_lib/Frames and Transforms/Rigid Transform  TranslationMethod=StandardAxis  TranslationLengthUnit=m  TranslationStandardAxis=+Y  TranslationStandardOffset=TNO_Veh_PARAM.Suspension.RA.Roll.Height  TranslationCartesianOffset=[0 0.05 0]  TranslationROffset=0  TranslationROffsetUnits=m  TranslationZOffset=0  TranslationZOffsetUnits=m  TranslationThetaOffset=0  TranslationThetaOffsetUnits=deg  RotationMethod=StandardAxis  RotationAngleUnits=deg  RotationStandardAxis=+Y  RotationAngle=90  RotationArbitraryAxis=[0 0 1]  FollAlignAxisA=+X  BaseAlignAxisA=+Y  FollAlignAxisB=+Y  BaseAlignAxisB=+Z  BlockFunction=simmechanics.library.frames_transforms.rigid_transform
  Body : PMIOPort  Port=1  Side=Left
  RA : PMIOPort  Port=2  Side=Right
  connections:
  RA/RConn1 -- Transform (RA)/RConn1
  Transform (Body)/LConn1 -- Axle Ctr/RConn1 -- Transform (RA)/LConn1
  Transform (Body)/RConn1 -- Body/RConn1

== system Vehicle_Dynamics_Tests/RHeave ==
  PS-Simulink Converter14 : nesl_utility/PS-Simulink Converter  PhysicalDomain=network_engine_domain  SubClassName=ps_output  LeftPortType=input  RightPortType=output  PseudoPeriodic=off  Frequencies=[]  Unit=m  AffineConversion=off
  To Workspace4 : ToWorkspace  VariableName=RAheave  SampleTime=-1
  Conn1 : PMIOPort  Port=1  Side=Left
  wires:
  PS-Simulink Converter14/1 -> To Workspace4/1
  connections:
  Conn1/RConn1 -- PS-Simulink Converter14/LConn1

== system Vehicle_Dynamics_Tests/RRoll ==
  PS-Simulink Converter16 : nesl_utility/PS-Simulink Converter  PhysicalDomain=network_engine_domain  SubClassName=ps_output  LeftPortType=input  RightPortType=output  PseudoPeriodic=off  Frequencies=[]  Unit=deg  AffineConversion=off
  To Workspace2 : ToWorkspace  VariableName=RAroll  SampleTime=-1
  Conn1 : PMIOPort  Port=1  Side=Right
  wires:
  PS-Simulink Converter16/1 -> To Workspace2/1
  connections:
  Conn1/RConn1 -- PS-Simulink Converter16/LConn1
